simulink model "ex4_10"  (R2020b)
settings: Solver=VariableStepAuto  StartTime=0.0  StopTime=10.0  RelTol=1e-3
libraries: dsparch4 x1
settings Model: Creator=seojoon  LastModifiedBy=seojoon

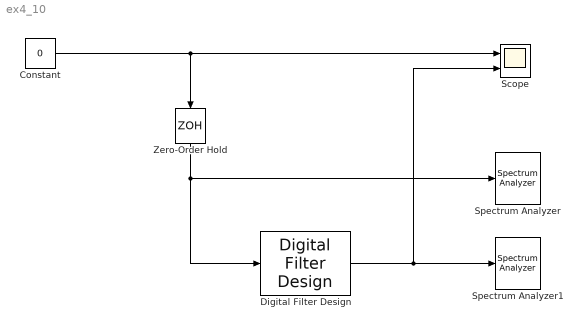
== system ex4_10 ==
  Constant : Constant  Value=0
  Digital Filter Design : dsparch4/Digital Filter Design  mwdsp_browser_bugfix_var=off
  Scope : Scope  NumInputPorts=2
  Spectrum Analyzer : SpectrumAnalyzer
  Spectrum Analyzer1 : SpectrumAnalyzer
  Zero-Order Hold : ZeroOrderHold  SampleTime=-1
  wires:
  Digital Filter Design/1 -> Scope/2, Spectrum Analyzer1/1
  Zero-Order Hold/1 -> Spectrum Analyzer/1, Digital Filter Design/1
  Constant/1 -> Scope/1, Zero-Order Hold/1
